simulink model "ergasia2ASK"  (R2021b)
settings: Solver=VariableStepAuto  StartTime=0.0  StopTime=1000  RelTol=1e-3
libraries: commchan3 x1, commrandsrc3 x1, dsparch4 x1
settings Model: Creator=giannis  LastModifiedBy=mluser
settings SolverCC: AlgebraicLoopSolver=TrustRegion
settings DebuggingCC: SFMachineParentedDataDiag=warning
settings SFSimCC: CustomCodeUndefinedFunction=UseInterfaceOnly

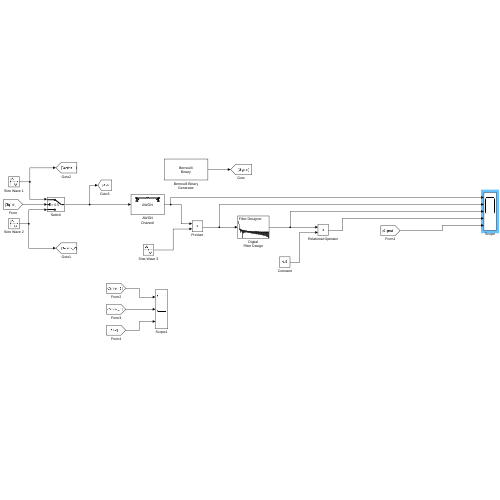
[thumbnail: Simulink's stored preview of the top-level diagram]
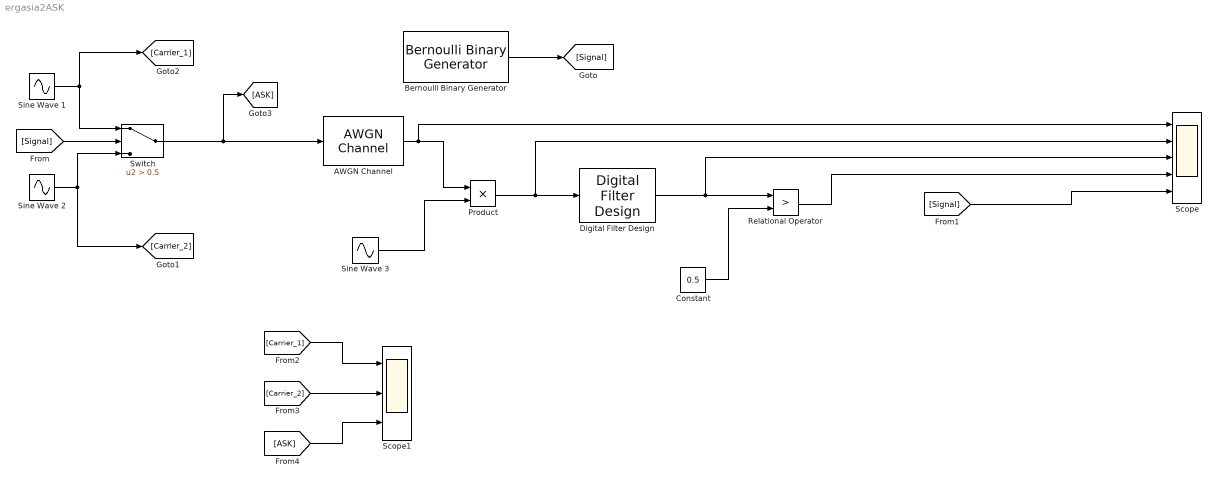
== system ergasia2ASK ==
  AWGN Channel : commchan3/AWGN Channel  InputProcessing=Columns as channels (frame based)  seed=81  noiseMode="Signal to noise ratio  (SNR)"  EbNodB=-24  EsNodB=10  SNRdB=-24  bitsPerSym=1  Ps=1  Tsym=5  variance=1
  Bernoulli Binary Generator : commrandsrc3/Bernoulli Binary Generator  ProbabilityOfZero=0.4  SeedSource=Parameter  Seed=81  SampleTime=5  SamplesPerFrame=1  OutputDataType=double  SimulateUsing=Interpreted execution
  Constant : Constant  Value=0.5
  Digital Filter Design : dsparch4/Digital Filter Design  mwdsp_browser_bugfix_var=off
  Product : Product  RndMeth=Zero
  Relational Operator : RelationalOperator  Operator=>  OutDataTypeStr='double'  RndMeth=Simplest
  Scope : Scope  NumInputPorts=5
  Scope1 : Scope  NumInputPorts=3
  Sine Wave 1 : Sin  SineType=Sample based  Amplitude=2  Samples=50  SampleTime=1/20
  Sine Wave 2 : Sin  SineType=Sample based  Amplitude=0.5  Samples=50  SampleTime=1/20
  Sine Wave 3 : Sin  SineType=Sample based  Samples=50  SampleTime=1/20
  Switch : Switch  Criteria=u2 > Threshold  Threshold=0.5
  wires:
  Sine Wave 1/1 -> [Carrier_1], Switch/1
  [Signal] -> Switch/2
  Sine Wave 2/1 -> [Carrier_2], Switch/3
  Switch/1 -> [ASK], AWGN Channel/1
  AWGN Channel/1 -> Scope/1, Product/1
  Sine Wave 3/1 -> Product/2
  Product/1 -> Scope/2, Digital Filter Design/1
  Digital Filter Design/1 -> Scope/3, Relational Operator/1
  Relational Operator/1 -> Scope/4
  [Signal] -> Scope/5
  Constant/1 -> Relational Operator/2
  [Carrier_1] -> Scope1/1
  [Carrier_2] -> Scope1/2
  [ASK] -> Scope1/3
  Bernoulli Binary Generator/1 -> [Signal]
